simulink model "tumbling_sim_v2"  (R2018a)
settings: Solver=VariableStepAuto  StartTime=0.0  StopTime=10
values from neighbouring files (symbols this model uses):
  omega0 = [1 -1 0.5]'    [init_tumbling.m]
  q0 = [0.8034 0.1600 0.4272 0.3828]'    [init_tumbling.m]
settings Model: Creator=abinalexpothen  LastModifiedBy=abinalexpothen

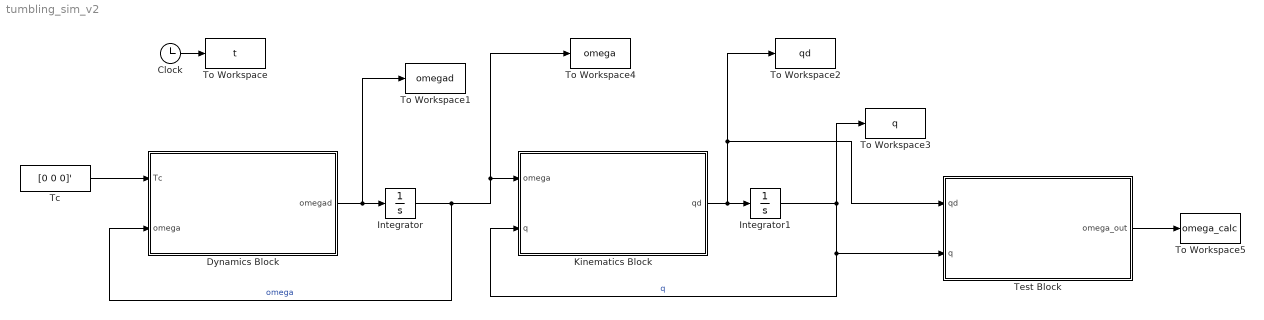
== system tumbling_sim_v2 ==
  Clock : Clock
  Dynamics Block : MATLAB Function  TreatAsAtomicUnit=on
  Integrator : Integrator  InitialCondition=omega0
  Integrator1 : Integrator  InitialCondition=q0
  Kinematics Block : MATLAB Function  TreatAsAtomicUnit=on
  Tc : Constant  Value=[0 0 0]'
  Test Block : MATLAB Function  TreatAsAtomicUnit=on
  To Workspace : ToWorkspace  VariableName=t  SampleTime=-1
  To Workspace1 : ToWorkspace  VariableName=omegad  SampleTime=-1
  To Workspace2 : ToWorkspace  VariableName=qd  SampleTime=-1
  To Workspace3 : ToWorkspace  VariableName=q  SampleTime=-1
  To Workspace4 : ToWorkspace  VariableName=omega  SampleTime=-1
  To Workspace5 : ToWorkspace  VariableName=omega_calc  SampleTime=-1
  wires:
  Clock/1 -> To Workspace/1
  Dynamics Block/1(omegad) -> To Workspace1/1, Integrator/1
  Integrator/1 -> Dynamics Block/2(omega), Kinematics Block/1(omega), To Workspace4/1  "omega"
  Kinematics Block/1(qd) -> Test Block/1(qd), To Workspace2/1, Integrator1/1
  Integrator1/1 -> To Workspace3/1, Test Block/2(q), Kinematics Block/2(q)  "q"
  Tc/1 -> Dynamics Block/1(Tc)
  Test Block/1(omega_out) -> To Workspace5/1

== matlab function tumbling_sim_v2/Kinematics Block ==
  data: omega input; q input; qd output
function qd = tumbling_kinematics(omega, q)

Omega = [0 -omega(1) -omega(2) -omega(3);
         omega(1) 0 omega(3) -omega(2);
         omega(2) -omega(3) 0 omega(1);
         omega(3) omega(2) -omega(1) 0];

qd = 0.5*Omega*q;

== matlab function tumbling_sim_v2/Dynamics Block ==
  data: Tc input; omegad output; omega input; J parameter
function omegad = tumbling_dynamics(Tc, omega, J)

omegad = J\(Tc-cross(omega,J*omega));

== matlab function tumbling_sim_v2/Test Block ==
  data: qd input; q input; omega_out output
function omega_out = test_block(qd, q)

H = 2*[-q(2) q(1) q(4) -q(3);
       -q(3) -q(4) q(1) q(2);
       -q(4) q(3) -q(2) q(1)];

omega_out = H*qd;
